simulink library "Blocks"  (R2022b)
settings: Solver=VariableStepAuto  StartTime=0.0  StopTime=10.0  RelTol=1e-3
undefined symbols (not defined in the file): h_send, h_stream_mocap, ID, Payload
libraries: uavmavlinklib x19, dspnetwork x9, hdlsllib x6, $bdroot x6, robotcorelib x2, etargetslib x1, slrealtimeiplib x1
settings Model: Creator=dsor  LastModifiedBy=dsor

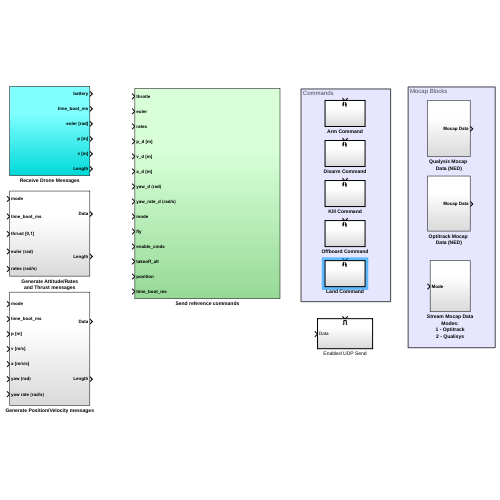
[thumbnail: Simulink's stored preview of the top-level diagram]
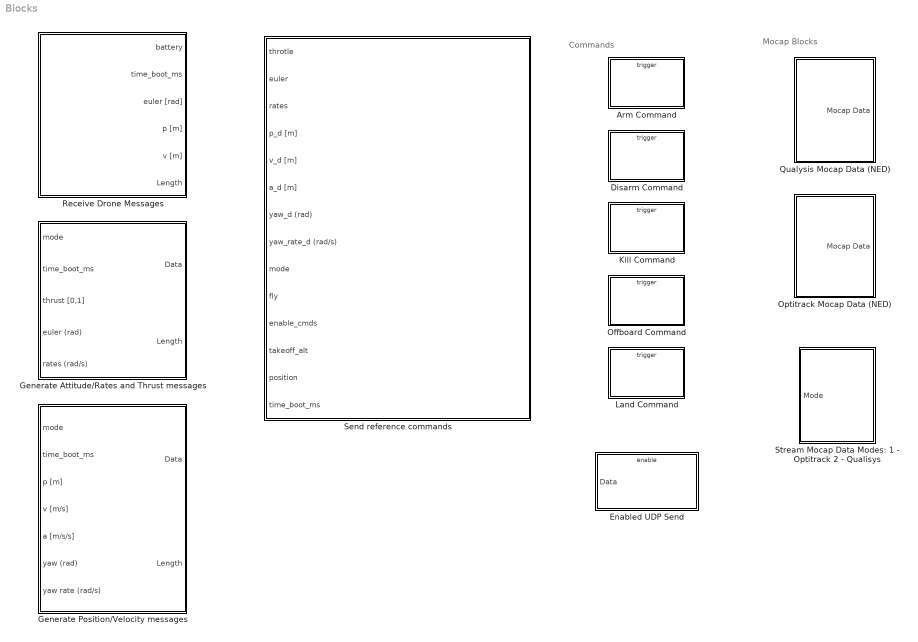
== system Blocks ==
  note: Commands
  note: Mocap Blocks
  Arm Command : Subsystem
  Disarm Command : Subsystem
  Enabled UDP Send : Subsystem
  Generate Attitude/Rates and Thrust messages : Subsystem
  Generate Position/Velocity messages : Subsystem
  Kill Command : Subsystem
  Land Command : Subsystem
  Offboard Command : Subsystem
  Optitrack Mocap Data (NED) : Subsystem
  Qualysis Mocap Data (NED) : Subsystem
  Receive Drone Messages : Subsystem
  Send reference commands : Subsystem
  Stream Mocap Data Modes: 1 - Optitrack 2 - Qualisys : Subsystem

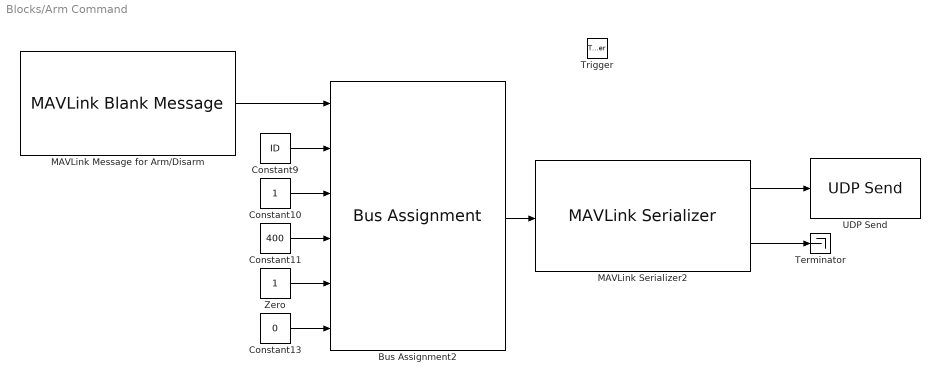
== system Blocks/Arm Command ==
  Trigger : TriggerPort  TriggerType=either  VariantControl=(inherit)  PortDimensions=1
  Bus Assignment2 : BusAssignment  AssignedSignals=Payload.target_system,Payload.target_component,Payload.command,Payload.param1,Payload.param2
  Constant10 : Constant  OutDataTypeStr=uint8
  Constant11 : Constant  Value=400  OutDataTypeStr=uint16
  Constant13 : Constant  Value=0  OutDataTypeStr=single
  Constant9 : Constant  Value=ID  OutDataTypeStr=uint8
  MAVLink Message for Arm/Disarm : uavmavlinklib/MAVLink Blank Message  dialectSource=Select from standard MAVLink dialects  dialect=common.xml  dialectCustom=common.xml  version=2  messageType=COMMAND_LONG  SystemID=255  ComponentID=240  SampleTime=-1
  MAVLink Serializer2 : uavmavlinklib/MAVLink Serializer  dialectSource=Select from standard MAVLink dialects  dialect=common.xml  dialectCustom=common.xml  version=2  messageType=COMMAND_LONG
  Terminator : Terminator
  UDP Send : dspnetwork/UDP Send  remoteURL=Remote_IP  remotePort=Remote_Port  localURL='0.0.0.0'  localPortSource=Specify via dialog  localPort=Local_Port  sendBufferSize=8192  sampletime=-1  blockPlatform=HOST  separateLengthPort=0
      settings: LibrarySourceBlock=embeddedtargetslib/Host Communication/UDP Send
  Zero : Constant  OutDataTypeStr=single
  wires:
  Zero/1 -> Bus Assignment2/5
  MAVLink Serializer2/1 -> UDP Send/1
  MAVLink Message for Arm/Disarm/1 -> Bus Assignment2/1
  Constant9/1 -> Bus Assignment2/2
  Constant13/1 -> Bus Assignment2/6
  Bus Assignment2/1 -> MAVLink Serializer2/1
  Constant10/1 -> Bus Assignment2/3
  Constant11/1 -> Bus Assignment2/4
  MAVLink Serializer2/2 -> Terminator/1

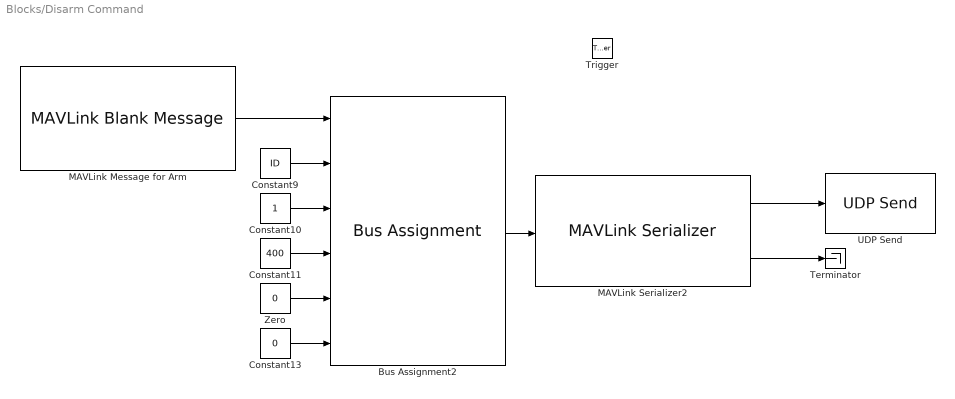
== system Blocks/Disarm Command ==
  Trigger : TriggerPort  TriggerType=either  VariantControl=(inherit)  PortDimensions=1
  Bus Assignment2 : BusAssignment  AssignedSignals=Payload.target_system,Payload.target_component,Payload.command,Payload.param1,Payload.param2
  Constant10 : Constant  OutDataTypeStr=uint8
  Constant11 : Constant  Value=400  OutDataTypeStr=uint16
  Constant13 : Constant  Value=0  OutDataTypeStr=single
  Constant9 : Constant  Value=ID  OutDataTypeStr=uint8
  MAVLink Message for Arm : uavmavlinklib/MAVLink Blank Message  dialectSource=Select from standard MAVLink dialects  dialect=common.xml  dialectCustom=common.xml  version=2  messageType=COMMAND_LONG  SystemID=255  ComponentID=240  SampleTime=-1
  MAVLink Serializer2 : uavmavlinklib/MAVLink Serializer  dialectSource=Select from standard MAVLink dialects  dialect=common.xml  dialectCustom=common.xml  version=2  messageType=COMMAND_LONG
  Terminator : Terminator
  UDP Send : dspnetwork/UDP Send  remoteURL=Remote_IP  remotePort=Remote_Port  localURL='0.0.0.0'  localPortSource=Specify via dialog  localPort=Local_Port  sendBufferSize=8192  sampletime=-1  blockPlatform=HOST  separateLengthPort=0
      settings: LibrarySourceBlock=embeddedtargetslib/Host Communication/UDP Send
  Zero : Constant  Value=0  OutDataTypeStr=single
  wires:
  Zero/1 -> Bus Assignment2/5
  MAVLink Message for Arm/1 -> Bus Assignment2/1
  Constant9/1 -> Bus Assignment2/2
  Constant13/1 -> Bus Assignment2/6
  Bus Assignment2/1 -> MAVLink Serializer2/1
  Constant10/1 -> Bus Assignment2/3
  Constant11/1 -> Bus Assignment2/4
  MAVLink Serializer2/1 -> UDP Send/1
  MAVLink Serializer2/2 -> Terminator/1

== system Blocks/Enabled UDP Send ==
  Data : Inport
  Enable : EnablePort
  UDP Send : dspnetwork/UDP Send  remoteURL=Remote_IP  remotePort=Remote_Port  localURL='0.0.0.0'  localPortSource=Specify via dialog  localPort=Local_Port  sendBufferSize=8192  sampletime=-1  blockPlatform=HOST  separateLengthPort=0
      settings: LibrarySourceBlock=embeddedtargetslib/Host Communication/UDP Send
  wires:
  Data/1 -> UDP Send/1

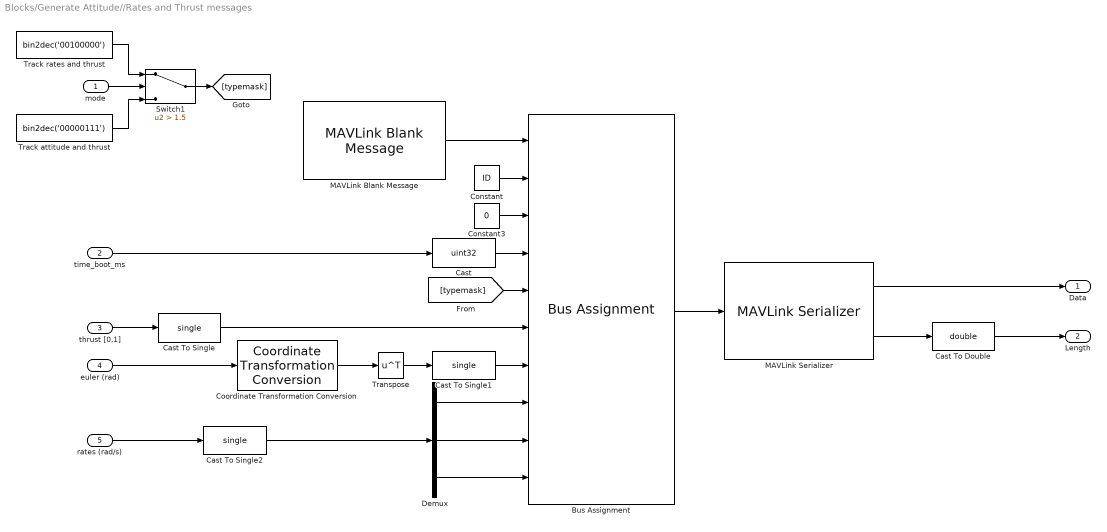
== system Blocks/Generate Attitude//Rates and Thrust messages ==
  mode : Inport  SampleTime=h_send
  time_boot_ms : Inport  Port=2  SampleTime=h_send
  thrust [0,1] : Inport  Port=3  SampleTime=h_send
  euler (rad) : Inport  Port=4  SampleTime=h_send
  rates (rad/s) : Inport  Port=5  SampleTime=h_send
  Bus Assignment : BusAssignment  AssignedSignals=Payload.target_system,Payload.target_component,Payload.time_boot_ms,Payload.type_mask,Payload.thrust,Payload.q,Payload.body_roll_rate,Payload.body_pitch_rate,Payload.body_yaw_rate
  Cast : DataTypeConversion  OutDataTypeStr=uint32  SaturateOnIntegerOverflow=off  RndMeth=Floor
  Cast To Double : DataTypeConversion  OutDataTypeStr=double  SaturateOnIntegerOverflow=off  RndMeth=Floor
  Cast To Single : DataTypeConversion  OutDataTypeStr=single  SaturateOnIntegerOverflow=off  RndMeth=Floor
  Cast To Single1 : DataTypeConversion  OutDataTypeStr=single  SaturateOnIntegerOverflow=off  RndMeth=Floor
  Cast To Single2 : DataTypeConversion  OutDataTypeStr=single  SaturateOnIntegerOverflow=off  RndMeth=Floor
  Constant : Constant  Value=ID  OutDataTypeStr=uint8  SampleTime=h_send
  Constant3 : Constant  Value=0  OutDataTypeStr=uint8  SampleTime=h_send
  Coordinate Transformation Conversion : robotcorelib/Coordinate Transformation Conversion  InputRepresentation=Euler Angles  InputEulerSequence=ZYX  ShowTrVecInputPort=on  OutputRepresentation=Quaternion  OutputEulerSequence=ZYX  ShowTrVecOutputPort=on  SimulateUsing=Interpreted execution
  Demux : Demux  Outputs=3
  MAVLink Blank Message : uavmavlinklib/MAVLink Blank Message  dialectSource=Select from standard MAVLink dialects  dialect=common.xml  dialectCustom=common.xml  version=2  messageType=SET_ATTITUDE_TARGET  SystemID=255  ComponentID=240  SampleTime=h_send
  MAVLink Serializer : uavmavlinklib/MAVLink Serializer  dialectSource=Select from standard MAVLink dialects  dialect=common.xml  dialectCustom=common.xml  version=2  messageType=SET_ATTITUDE_TARGET
  Switch1 : Switch  Criteria=u2 > Threshold  Threshold=1.5  SaturateOnIntegerOverflow=off  InputSameDT=off
  Track attitude and thrust : Constant  Value=bin2dec('00000111')  OutDataTypeStr=uint8  SampleTime=h_send
  Track rates and thrust : Constant  Value=bin2dec('00100000')  OutDataTypeStr=uint8  SampleTime=h_send
  Transpose : Math  Operator=transpose
  Data : Outport  SampleTime=h_send
  Length : Outport  Port=2  SampleTime=h_send
  wires:
  time_boot_ms/1 -> Cast/1
  MAVLink Serializer/2 -> Cast To Double/1
  Cast/1 -> Bus Assignment/4
  Cast To Single1/1 -> Bus Assignment/7
  thrust [0,1]/1 -> Cast To Single/1
  [typemask] -> Bus Assignment/5
  Transpose/1 -> Cast To Single1/1
  Constant3/1 -> Bus Assignment/3
  Constant/1 -> Bus Assignment/2
  MAVLink Blank Message/1 -> Bus Assignment/1
  Cast To Single/1 -> Bus Assignment/6
  Bus Assignment/1 -> MAVLink Serializer/1
  Coordinate Transformation Conversion/1 -> Transpose/1
  euler (rad)/1 -> Coordinate Transformation Conversion/1
  rates (rad/s)/1 -> Cast To Single2/1
  Demux/1 -> Bus Assignment/8
  Demux/2 -> Bus Assignment/9
  Demux/3 -> Bus Assignment/10
  mode/1 -> Switch1/2
  Track rates and thrust/1 -> Switch1/1
  Track attitude and thrust/1 -> Switch1/3
  Switch1/1 -> [typemask]
  Cast To Single2/1 -> Demux/1
  MAVLink Serializer/1 -> Data/1
  Cast To Double/1 -> Length/1

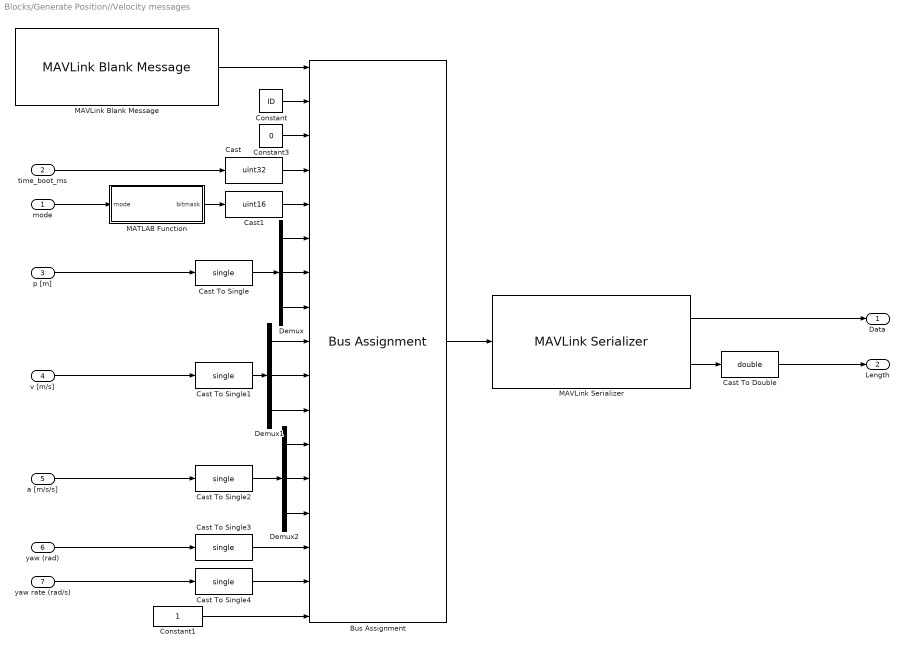
== system Blocks/Generate Position//Velocity messages ==
  mode : Inport  SampleTime=h_send
  time_boot_ms : Inport  Port=2  SampleTime=h_send
  p [m] : Inport  Port=3  SampleTime=h_send
  v [m/s] : Inport  Port=4  SampleTime=h_send
  a [m/s/s] : Inport  Port=5  SampleTime=h_send
  yaw (rad) : Inport  Port=6  SampleTime=h_send
  yaw rate (rad/s) : Inport  Port=7  SampleTime=h_send
  Bus Assignment : BusAssignment  AssignedSignals=Payload.target_system,Payload.target_component,Payload.time_boot_ms,Payload.type_mask,Payload.x,Payload.y,Payload.z,Payload.vx,Payload.vy,Payload.vz,Payload.afx,Payload.afy,Payload.afz,Payload.yaw,Payload.yaw_rate,Payload.coordinate_frame
  Cast : DataTypeConversion  OutDataTypeStr=uint32  SaturateOnIntegerOverflow=off  RndMeth=Floor
  Cast To Double : DataTypeConversion  OutDataTypeStr=double  SaturateOnIntegerOverflow=off  RndMeth=Floor
  Cast To Single{,1..4} (5 alike) : DataTypeConversion  OutDataTypeStr=single  SaturateOnIntegerOverflow=off  RndMeth=Floor
  Cast1 : DataTypeConversion  OutDataTypeStr=uint16  SaturateOnIntegerOverflow=off  RndMeth=Floor
  Constant : Constant  Value=ID  OutDataTypeStr=uint8  SampleTime=h_send
  Constant1 : Constant  OutDataTypeStr=uint8  SampleTime=h_send
  Constant3 : Constant  Value=0  OutDataTypeStr=uint8  SampleTime=h_send
  Demux : Demux  Outputs=3
  Demux1 : Demux  Outputs=3
  Demux2 : Demux  Outputs=3
  MATLAB Function : MATLAB Function  TreatAsAtomicUnit=on
  MAVLink Blank Message : uavmavlinklib/MAVLink Blank Message  dialectSource=Select from standard MAVLink dialects  dialect=common.xml  dialectCustom=common.xml  version=2  messageType=SET_POSITION_TARGET_LOCAL_NED  SystemID=255  ComponentID=240  SampleTime=h_send
  MAVLink Serializer : uavmavlinklib/MAVLink Serializer  dialectSource=Select from standard MAVLink dialects  dialect=common.xml  dialectCustom=common.xml  version=2  messageType=SET_POSITION_TARGET_LOCAL_NED
  Data : Outport  SampleTime=h_send
  Length : Outport  Port=2  SampleTime=h_send
  wires:
  Cast To Single4/1 -> Bus Assignment/16
  Cast1/1 -> Bus Assignment/5
  mode/1 -> MATLAB Function/1(mode)
  yaw rate (rad/s)/1 -> Cast To Single4/1
  Cast To Single3/1 -> Bus Assignment/15
  Cast To Single2/1 -> Demux2/1
  Cast To Single1/1 -> Demux1/1
  Cast To Single/1 -> Demux/1
  Constant1/1 -> Bus Assignment/17
  yaw (rad)/1 -> Cast To Single3/1
  Demux2/1 -> Bus Assignment/12
  Demux2/2 -> Bus Assignment/13
  Demux2/3 -> Bus Assignment/14
  a [m/s/s]/1 -> Cast To Single2/1
  v [m/s]/1 -> Cast To Single1/1
  Demux1/3 -> Bus Assignment/11
  Demux1/2 -> Bus Assignment/10
  Demux1/1 -> Bus Assignment/9
  p [m]/1 -> Cast To Single/1
  Demux/1 -> Bus Assignment/6
  Demux/2 -> Bus Assignment/7
  Demux/3 -> Bus Assignment/8
  Bus Assignment/1 -> MAVLink Serializer/1
  MAVLink Blank Message/1 -> Bus Assignment/1
  Constant/1 -> Bus Assignment/2
  Constant3/1 -> Bus Assignment/3
  MATLAB Function/1(bitmask) -> Cast1/1
  Cast/1 -> Bus Assignment/4
  MAVLink Serializer/2 -> Cast To Double/1
  time_boot_ms/1 -> Cast/1
  MAVLink Serializer/1 -> Data/1
  Cast To Double/1 -> Length/1

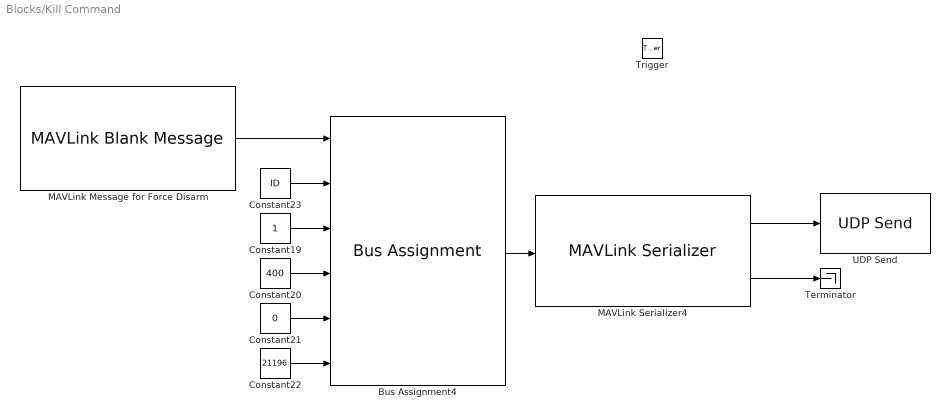
== system Blocks/Kill Command ==
  Trigger : TriggerPort  TriggerType=either  VariantControl=(inherit)  PortDimensions=1
  Bus Assignment4 : BusAssignment  AssignedSignals=Payload.target_system,Payload.target_component,Payload.command,Payload.param1,Payload.param2
  Constant19 : Constant  OutDataTypeStr=uint8
  Constant20 : Constant  Value=400  OutDataTypeStr=uint16
  Constant21 : Constant  Value=0  OutDataTypeStr=single
  Constant22 : Constant  Value=21196  OutDataTypeStr=single
  Constant23 : Constant  Value=ID  OutDataTypeStr=uint8
  MAVLink Message for Force Disarm : uavmavlinklib/MAVLink Blank Message  dialectSource=Select from standard MAVLink dialects  dialect=common.xml  dialectCustom=common.xml  version=2  messageType=COMMAND_LONG  SystemID=255  ComponentID=240  SampleTime=-1
  MAVLink Serializer4 : uavmavlinklib/MAVLink Serializer  dialectSource=Select from standard MAVLink dialects  dialect=common.xml  dialectCustom=common.xml  version=2  messageType=COMMAND_LONG
  Terminator : Terminator
  UDP Send : dspnetwork/UDP Send  remoteURL=Remote_IP  remotePort=Remote_Port  localURL='0.0.0.0'  localPortSource=Specify via dialog  localPort=Local_Port  sendBufferSize=8192  sampletime=-1  blockPlatform=HOST  separateLengthPort=0
      settings: LibrarySourceBlock=embeddedtargetslib/Host Communication/UDP Send
  wires:
  Constant20/1 -> Bus Assignment4/4
  Constant22/1 -> Bus Assignment4/6
  Constant21/1 -> Bus Assignment4/5
  MAVLink Message for Force Disarm/1 -> Bus Assignment4/1
  Bus Assignment4/1 -> MAVLink Serializer4/1
  Constant19/1 -> Bus Assignment4/3
  Constant23/1 -> Bus Assignment4/2
  MAVLink Serializer4/1 -> UDP Send/1
  MAVLink Serializer4/2 -> Terminator/1

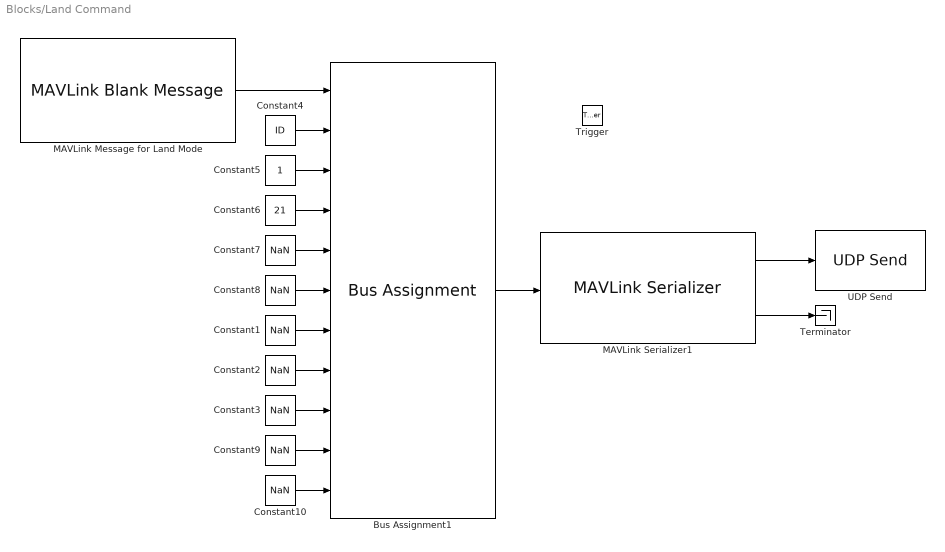
== system Blocks/Land Command ==
  Trigger : TriggerPort  VariantControl=(inherit)  PortDimensions=1
  Bus Assignment1 : BusAssignment  AssignedSignals=Payload.target_system,Payload.target_component,Payload.command,Payload.param1,Payload.param2,Payload.param3,Payload.param4,Payload.param5,Payload.param6,Payload.param7
  Constant{1..3,7..10} (7 alike) : Constant  Value=NaN  OutDataTypeStr=single
  Constant4 : Constant  Value=ID  OutDataTypeStr=uint8
  Constant5 : Constant  OutDataTypeStr=uint8
  Constant6 : Constant  Value=21  OutDataTypeStr=uint16
  MAVLink Message for Land Mode : uavmavlinklib/MAVLink Blank Message  dialectSource=Select from standard MAVLink dialects  dialect=common.xml  dialectCustom=common.xml  version=2  messageType=COMMAND_LONG  SystemID=255  ComponentID=240  SampleTime=-1
  MAVLink Serializer1 : uavmavlinklib/MAVLink Serializer  dialectSource=Select from standard MAVLink dialects  dialect=common.xml  dialectCustom=common.xml  version=2  messageType=COMMAND_LONG
  Terminator : Terminator
  UDP Send : dspnetwork/UDP Send  remoteURL=Remote_IP  remotePort=Remote_Port  localURL='0.0.0.0'  localPortSource=Specify via dialog  localPort=Local_Port  sendBufferSize=8192  sampletime=-1  blockPlatform=HOST  separateLengthPort=0
      settings: LibrarySourceBlock=embeddedtargetslib/Host Communication/UDP Send
  wires:
  Constant4/1 -> Bus Assignment1/2
  Constant8/1 -> Bus Assignment1/6
  Constant6/1 -> Bus Assignment1/4
  Constant5/1 -> Bus Assignment1/3
  MAVLink Message for Land Mode/1 -> Bus Assignment1/1
  Bus Assignment1/1 -> MAVLink Serializer1/1
  Constant7/1 -> Bus Assignment1/5
  Constant10/1 -> Bus Assignment1/11
  Constant9/1 -> Bus Assignment1/10
  Constant3/1 -> Bus Assignment1/9
  Constant2/1 -> Bus Assignment1/8
  Constant1/1 -> Bus Assignment1/7
  MAVLink Serializer1/1 -> UDP Send/1
  MAVLink Serializer1/2 -> Terminator/1

== system Blocks/Offboard Command ==
  Trigger : TriggerPort  TriggerType=either  VariantControl=(inherit)  PortDimensions=1
  Bus Assignment1 : BusAssignment  AssignedSignals=Payload.target_system,Payload.target_component,Payload.command,Payload.param1,Payload.param2
  Constant4 : Constant  Value=ID  OutDataTypeStr=uint8
  Constant5 : Constant  OutDataTypeStr=uint8
  Constant6 : Constant  Value=176  OutDataTypeStr=uint16
  Constant7 : Constant  OutDataTypeStr=single
  Constant8 : Constant  Value=6  OutDataTypeStr=single
  MAVLink Message for Offboard Mode : uavmavlinklib/MAVLink Blank Message  dialectSource=Select from standard MAVLink dialects  dialect=common.xml  dialectCustom=common.xml  version=2  messageType=COMMAND_LONG  SystemID=255  ComponentID=240  SampleTime=-1
  MAVLink Serializer1 : uavmavlinklib/MAVLink Serializer  dialectSource=Select from standard MAVLink dialects  dialect=common.xml  dialectCustom=common.xml  version=2  messageType=COMMAND_LONG
  Terminator : Terminator
  UDP Send : dspnetwork/UDP Send  remoteURL=Remote_IP  remotePort=Remote_Port  localURL='0.0.0.0'  localPortSource=Specify via dialog  localPort=Local_Port  sendBufferSize=8192  sampletime=-1  blockPlatform=HOST  separateLengthPort=0
      settings: LibrarySourceBlock=embeddedtargetslib/Host Communication/UDP Send
  wires:
  Constant7/1 -> Bus Assignment1/5
  Bus Assignment1/1 -> MAVLink Serializer1/1
  MAVLink Message for Offboard Mode/1 -> Bus Assignment1/1
  Constant5/1 -> Bus Assignment1/3
  Constant6/1 -> Bus Assignment1/4
  Constant8/1 -> Bus Assignment1/6
  Constant4/1 -> Bus Assignment1/2
  MAVLink Serializer1/1 -> UDP Send/1
  MAVLink Serializer1/2 -> Terminator/1

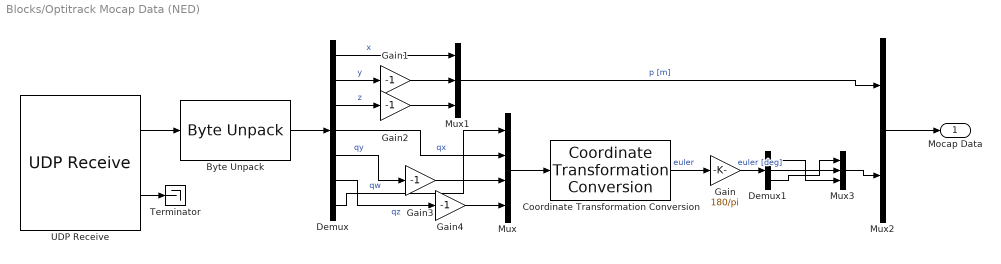
== system Blocks/Optitrack Mocap Data (NED) ==
  Byte Unpack : etargetslib/Byte Unpack  dimensions={[7]}  datatypes={'double'}  byteAlign=4
  Coordinate Transformation Conversion : robotcorelib/Coordinate Transformation Conversion  InputRepresentation=Quaternion  InputEulerSequence=ZYX  ShowTrVecInputPort=on  OutputRepresentation=Euler Angles  OutputEulerSequence=ZYX  ShowTrVecOutputPort=on  SimulateUsing=Interpreted execution
  Demux : Demux  Outputs=7
  Demux1 : Demux  Outputs=3
  Gain : Gain  Gain=180/pi
  Gain{1..4} (4 alike) : Gain  Gain=-1
  Mux : Mux
  Mux1 : Mux  Inputs=3
  Mux2 : Mux  Inputs=2
  Mux3 : Mux  Inputs=3
  Terminator : Terminator
  UDP Receive : dspnetwork/UDP Receive  localURL='0.0.0.0'  localPort=5000  remoteURL='0.0.0.0'  remotePort=-1  recvBufferSize=56  dims=56  signalDatatype=uint8  isComplex=off  isVarSize=off  showBlockingTime=on  blockingTime=0  sampletime=h_optitrack  blockPlatform=HOST
  Mocap Data : Outport
  wires:
  Mux3/1 -> Mux2/2
  Demux1/2 -> Mux3/2
  Demux1/1 -> Mux3/3
  Demux1/3 -> Mux3/1
  Gain/1 -> Demux1/1  "euler [deg]"
  Gain4/1 -> Mux/4
  Gain3/1 -> Mux/3
  Gain2/1 -> Mux1/3
  Gain1/1 -> Mux1/2
  UDP Receive/1 -> Byte Unpack/1
  Demux/3 -> Gain2/1  "z"
  Byte Unpack/1 -> Demux/1
  Demux/1 -> Mux1/1  "x"
  Demux/2 -> Gain1/1  "y"
  UDP Receive/2 -> Terminator/1
  Mux/1 -> Coordinate Transformation Conversion/1
  Mux1/1 -> Mux2/1  "p [m]"
  Mux2/1 -> Mocap Data/1
  Coordinate Transformation Conversion/1 -> Gain/1  "euler"
  Demux/7 -> Mux/1  "qw"
  Demux/4 -> Mux/2  "qx"
  Demux/5 -> Gain3/1  "qy"
  Demux/6 -> Gain4/1  "qz"

== system Blocks/Qualysis Mocap Data (NED) ==
  Constant1 : Constant
  Gain{6..7,9..10} (4 alike) : Gain  Gain=-1
  Mux : Mux  Inputs=6
  Subsystem : Subsystem
  Terminator : Terminator
  UDP Receive1 : dspnetwork/UDP Receive  localURL='0.0.0.0'  localPort=9089  remoteURL='0.0.0.0'  remotePort=-1  recvBufferSize=64  dims=255  signalDatatype=uint8  isComplex=off  isVarSize=off  showBlockingTime=on  blockingTime=0  sampletime=h_qualisys  blockPlatform=HOST
      settings: LibrarySourceBlock=embeddedtargetslib/Host Communication/UDP Receive
  Mocap Data : Outport
  wires:
  Gain6/1 -> Mux/5
  UDP Receive1/2 -> Terminator/1
  Constant1/1 -> Subsystem/2(Object number)
  Subsystem/3(z [m]) -> Gain10/1
  Subsystem/2(y [m]) -> Gain9/1
  UDP Receive1/1 -> Subsystem/1(Data)
  Subsystem/5(pitch [deg]) -> Gain6/1
  Subsystem/6(yaw [deg]) -> Gain7/1
  Gain7/1 -> Mux/6
  Gain10/1 -> Mux/3
  Gain9/1 -> Mux/2
  Subsystem/1(x [m]) -> Mux/1
  Subsystem/4(roll [deg]) -> Mux/4
  Mux/1 -> Mocap Data/1

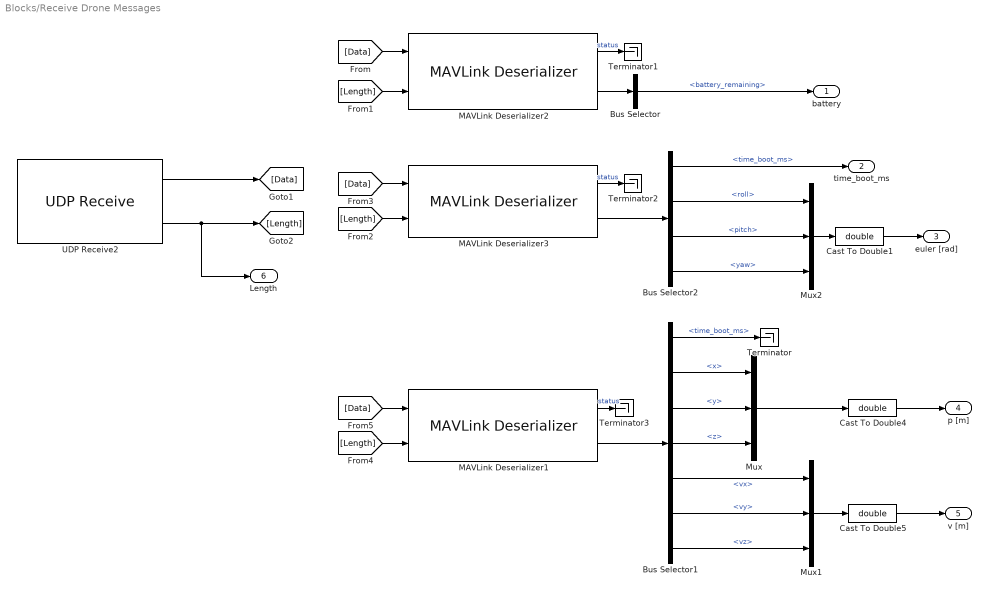
== system Blocks/Receive Drone Messages ==
  Bus Selector : BusSelector  OutputSignals=Payload.battery_remaining
  Bus Selector1 : BusSelector  OutputSignals=Payload.time_boot_ms,Payload.x,Payload.y,Payload.z,Payload.vx,Payload.vy,Payload.vz
  Bus Selector2 : BusSelector  OutputSignals=Payload.time_boot_ms,Payload.roll,Payload.pitch,Payload.yaw
  Cast To Double1 : DataTypeConversion  OutDataTypeStr=double  SaturateOnIntegerOverflow=off  RndMeth=Floor
  Cast To Double4 : DataTypeConversion  OutDataTypeStr=double  SaturateOnIntegerOverflow=off  RndMeth=Floor
  Cast To Double5 : DataTypeConversion  OutDataTypeStr=double  SaturateOnIntegerOverflow=off  RndMeth=Floor
  MAVLink Deserializer1 : uavmavlinklib/MAVLink Deserializer  dialectSource=Select from standard MAVLink dialects  dialect=common.xml  dialectCustom=common.xml  version=2  messageType=LOCAL_POSITION_NED  inputDataLength=on  SystemIDFilter=off  systemID=1  ComponentIDFilter=off  componentID=1  queueMsg=off  queueMsgSize=50  dropNum=off
  MAVLink Deserializer2 : uavmavlinklib/MAVLink Deserializer  dialectSource=Select from standard MAVLink dialects  dialect=common.xml  dialectCustom=common.xml  version=2  messageType=SYS_STATUS  inputDataLength=on  SystemIDFilter=off  systemID=1  ComponentIDFilter=off  componentID=1  queueMsg=off  queueMsgSize=50  dropNum=off
  MAVLink Deserializer3 : uavmavlinklib/MAVLink Deserializer  dialectSource=Select from standard MAVLink dialects  dialect=common.xml  dialectCustom=common.xml  version=2  messageType=ATTITUDE  inputDataLength=on  SystemIDFilter=off  systemID=1  ComponentIDFilter=off  componentID=1  queueMsg=off  queueMsgSize=50  dropNum=off
  Mux : Mux  Inputs=3
  Mux1 : Mux  Inputs=3
  Mux2 : Mux  Inputs=3
  Terminator{,1..3} (4 alike) : Terminator
  UDP Receive2 : dspnetwork/UDP Receive  localURL='0.0.0.0'  localPort=Local_Port  remoteURL='0.0.0.0'  remotePort=-1  recvBufferSize=8192  dims=255  signalDatatype=uint8  isComplex=off  isVarSize=off  showBlockingTime=on  blockingTime=0  sampletime=h_receive  blockPlatform=HOST
      settings: LibrarySourceBlock=embeddedtargetslib/Host Communication/UDP Receive
  battery : Outport
  time_boot_ms : Outport  Port=2
  euler [rad] : Outport  Port=3
  p [m] : Outport  Port=4
  v [m] : Outport  Port=5
  Length : Outport  Port=6
  wires:
  Mux1/1 -> Cast To Double5/1
  Cast To Double4/1 -> p [m]/1
  [Length] -> MAVLink Deserializer1/2
  Cast To Double5/1 -> v [m]/1
  Bus Selector1/6 -> Mux1/2  "<vy>"
  Bus Selector1/3 -> Mux/2  "<y>"
  Bus Selector1/1 -> Terminator/1  "<time_boot_ms>"
  Mux/1 -> Cast To Double4/1
  [Length] -> MAVLink Deserializer3/2
  Bus Selector1/2 -> Mux/1  "<x>"
  Bus Selector2/1 -> time_boot_ms/1  "<time_boot_ms>"
  [Data] -> MAVLink Deserializer3/1
  MAVLink Deserializer1/2 -> Bus Selector1/1
  Bus Selector1/7 -> Mux1/3  "<vz>"
  Bus Selector/1 -> battery/1  "<battery_remaining>"
  [Data] -> MAVLink Deserializer1/1
  [Data] -> MAVLink Deserializer2/1
  Bus Selector2/2 -> Mux2/1  "<roll>"
  Mux2/1 -> Cast To Double1/1
  MAVLink Deserializer1/1 -> Terminator3/1  "status"
  Bus Selector2/4 -> Mux2/3  "<yaw>"
  Bus Selector1/5 -> Mux1/1  "<vx>"
  Bus Selector2/3 -> Mux2/2  "<pitch>"
  MAVLink Deserializer2/1 -> Terminator1/1  "status"
  [Length] -> MAVLink Deserializer2/2
  MAVLink Deserializer3/2 -> Bus Selector2/1
  Bus Selector1/4 -> Mux/3  "<z>"
  MAVLink Deserializer2/2 -> Bus Selector/1
  Cast To Double1/1 -> euler [rad]/1
  MAVLink Deserializer3/1 -> Terminator2/1  "status"
  UDP Receive2/2 -> Length/1, [Length]
  UDP Receive2/1 -> [Data]

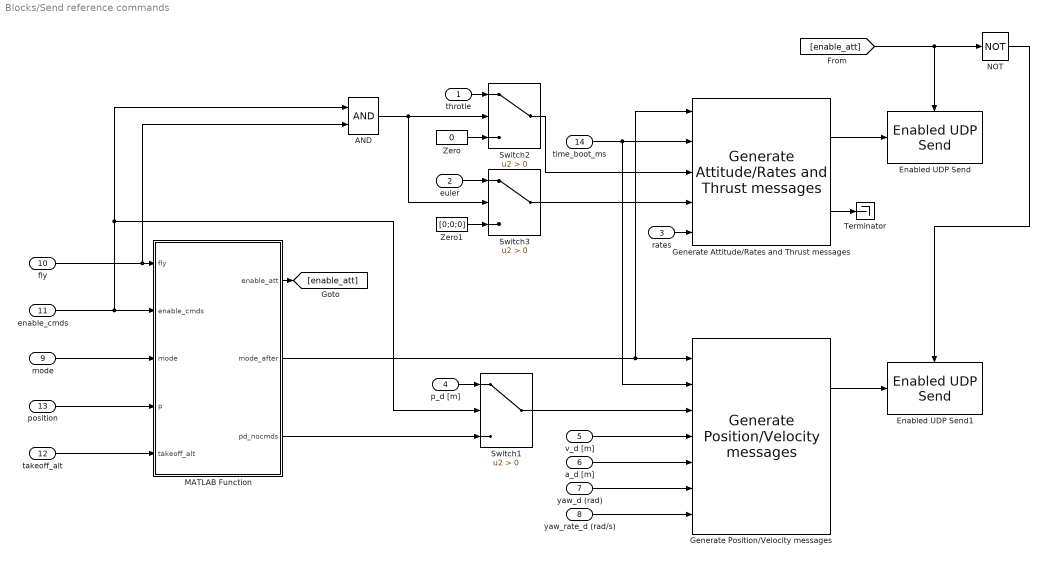
== system Blocks/Send reference commands ==
  throtle : Inport  SampleTime=h_send
  euler : Inport  Port=2  SampleTime=h_send
  rates : Inport  Port=3  SampleTime=h_send
  p_d [m] : Inport  Port=4  SampleTime=h_send
  v_d [m] : Inport  Port=5  SampleTime=h_send
  a_d [m] : Inport  Port=6  SampleTime=h_send
  yaw_d (rad) : Inport  Port=7  SampleTime=h_send
  yaw_rate_d (rad/s) : Inport  Port=8  SampleTime=h_send
  mode : Inport  Port=9  SampleTime=h_send
  fly : Inport  Port=10  SampleTime=h_send
  enable_cmds : Inport  Port=11  SampleTime=h_send
  takeoff_alt : Inport  Port=12  SampleTime=h_send
  position : Inport  Port=13  SampleTime=h_send
  time_boot_ms : Inport  Port=14  SampleTime=h_send
  AND : Logic  IconShape=distinctive  AllPortsSameDT=off  OutDataTypeStr=boolean
  Enabled UDP Send : $bdroot/Enabled UDP Send  SystemSampleTime=-1  VariantActivationTime=update diagram  Latency=0  AutoFrameSizeCalculation=off
  Enabled UDP Send1 : $bdroot/Enabled UDP Send  SystemSampleTime=-1  VariantActivationTime=update diagram  Latency=0  AutoFrameSizeCalculation=off
  Generate Attitude/Rates and Thrust messages : $bdroot/Generate Attitude//Rates and Thrust messages  SystemSampleTime=-1  VariantActivationTime=update diagram  Latency=0  AutoFrameSizeCalculation=off
  Generate Position/Velocity messages : $bdroot/Generate Position//Velocity messages  SystemSampleTime=-1  VariantActivationTime=update diagram  Latency=0  AutoFrameSizeCalculation=off
  MATLAB Function : MATLAB Function  TreatAsAtomicUnit=on
  NOT : Logic  Operator=NOT  IconShape=distinctive  AllPortsSameDT=off  OutDataTypeStr=boolean
  Switch1 : Switch  Criteria=u2 > Threshold  SaturateOnIntegerOverflow=off  InputSameDT=off
  Switch2 : Switch  Criteria=u2 > Threshold  SaturateOnIntegerOverflow=off  InputSameDT=off
  Switch3 : Switch  Criteria=u2 > Threshold  SaturateOnIntegerOverflow=off  InputSameDT=off
  Terminator : Terminator
  Zero : Constant  Value=0  OutDataTypeStr=Inherit: Inherit via back propagation
  Zero1 : Constant  Value=[0;0;0]  OutDataTypeStr=Inherit: Inherit via back propagation
  wires:
  v_d [m]/1 -> Generate Position/Velocity messages/4
  throtle/1 -> Switch2/1
  position/1 -> MATLAB Function/4(p)
  p_d [m]/1 -> Switch1/1
  Switch1/1 -> Generate Position/Velocity messages/3
  yaw_d (rad)/1 -> Generate Position/Velocity messages/6
  a_d [m]/1 -> Generate Position/Velocity messages/5
  Zero1/1 -> Switch3/3
  Switch3/1 -> Generate Attitude/Rates and Thrust messages/4
  enable_cmds/1 -> Switch1/2, AND/1, MATLAB Function/2(enable_cmds)
  MATLAB Function/2(mode_after) -> Generate Attitude/Rates and Thrust messages/1, Generate Position/Velocity messages/1
  Switch2/1 -> Generate Attitude/Rates and Thrust messages/3
  AND/1 -> Switch3/2, Switch2/2
  MATLAB Function/3(pd_nocmds) -> Switch1/3
  rates/1 -> Generate Attitude/Rates and Thrust messages/5
  yaw_rate_d (rad/s)/1 -> Generate Position/Velocity messages/7
  time_boot_ms/1 -> Generate Attitude/Rates and Thrust messages/2, Generate Position/Velocity messages/2
  fly/1 -> AND/2, MATLAB Function/1(fly)
  mode/1 -> MATLAB Function/3(mode)
  euler/1 -> Switch3/1
  Zero/1 -> Switch2/3
  takeoff_alt/1 -> MATLAB Function/5(takeoff_alt)
  Generate Attitude/Rates and Thrust messages/1 -> Enabled UDP Send/1
  Generate Attitude/Rates and Thrust messages/2 -> Terminator/1
  Generate Position/Velocity messages/1 -> Enabled UDP Send1/1
  MATLAB Function/1(enable_att) -> [enable_att]
  [enable_att] -> NOT/1, Enabled UDP Send/Enable
  NOT/1 -> Enabled UDP Send1/Enable

== system Blocks/Stream Mocap Data Modes: 1 - Optitrack 2 - Qualisys ==
  note: Modes
      | 0 - Disable
      | 1 - Optitrack
      | 2 - Qualisys
  Mode : Inport
  Optitrack Mocap Data (NED) : $bdroot/Optitrack Mocap  Data (NED)  SystemSampleTime=-1  VariantActivationTime=update diagram  Latency=0  AutoFrameSizeCalculation=off
  Qualysis Mocap Data (NED) : $bdroot/Qualysis Mocap  Data (NED)  SystemSampleTime=-1  VariantActivationTime=update diagram  Latency=0  AutoFrameSizeCalculation=off
  Rate Transition : RateTransition  OutPortSampleTime=h_stream_mocap
  Rate Transition1 : RateTransition  OutPortSampleTime=h_stream_mocap
  Stream Mocap Data to the Drone (must be in NED) : Subsystem
  Switch : Switch  Criteria=u2 > Threshold  Threshold=1.5  SaturateOnIntegerOverflow=off  InputSameDT=off
  wires:
  Switch/1 -> Stream Mocap Data to the Drone (must be in NED)/2(Mocap Data)
  Optitrack Mocap Data (NED)/1 -> Rate Transition1/1
  Qualysis Mocap Data (NED)/1 -> Rate Transition/1
  Rate Transition/1 -> Switch/1
  Mode/1 -> Stream Mocap Data to the Drone (must be in NED)/1(enable), Switch/2
  Rate Transition1/1 -> Switch/3

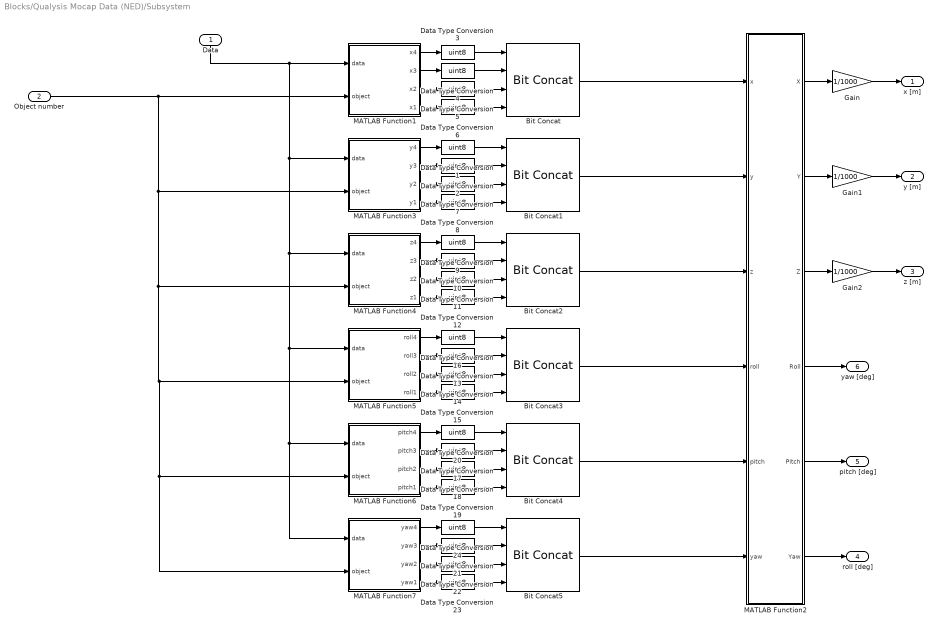
== system Blocks/Qualysis Mocap Data (NED)/Subsystem ==
  Data : Inport
  Object number : Inport  Port=2
  Bit Concat{,1..5} (6 alike) : hdlsllib/Logic and Bit Operations/Bit Concat  numInputs=4
  Data Type Conversion{1..24} (24 alike) : DataTypeConversion  OutDataTypeStr=uint8  SaturateOnIntegerOverflow=off  RndMeth=Floor
  Gain : Gain  Gain=1/1000
  Gain1 : Gain  Gain=1/1000
  Gain2 : Gain  Gain=1/1000
  MATLAB Function1 : MATLAB Function  TreatAsAtomicUnit=on
  MATLAB Function2 : MATLAB Function  TreatAsAtomicUnit=on
  MATLAB Function3 : MATLAB Function  TreatAsAtomicUnit=on
  MATLAB Function4 : MATLAB Function  TreatAsAtomicUnit=on
  MATLAB Function5 : MATLAB Function  TreatAsAtomicUnit=on
  MATLAB Function6 : MATLAB Function  TreatAsAtomicUnit=on
  MATLAB Function7 : MATLAB Function  TreatAsAtomicUnit=on
  x [m] : Outport  VectorParamsAs1DForOutWhenUnconnected=off
  y [m] : Outport  Port=2  VectorParamsAs1DForOutWhenUnconnected=off
  z [m] : Outport  Port=3  VectorParamsAs1DForOutWhenUnconnected=off
  roll [deg] : Outport  Port=4  VectorParamsAs1DForOutWhenUnconnected=off
  pitch [deg] : Outport  Port=5  VectorParamsAs1DForOutWhenUnconnected=off
  yaw [deg] : Outport  Port=6  VectorParamsAs1DForOutWhenUnconnected=off
  wires:
  Data Type Conversion6/1 -> Bit Concat/4
  Data Type Conversion3/1 -> Bit Concat/1
  MATLAB Function1/3(x2) -> Data Type Conversion5/1
  MATLAB Function2/1(X) -> Gain/1
  MATLAB Function4/1(z4) -> Data Type Conversion9/1
  MATLAB Function4/2(z3) -> Data Type Conversion10/1
  Bit Concat2/1 -> MATLAB Function2/3(z)
  Data Type Conversion12/1 -> Bit Concat2/4
  Data Type Conversion11/1 -> Bit Concat2/3
  MATLAB Function4/4(z1) -> Data Type Conversion12/1
  Data Type Conversion10/1 -> Bit Concat2/2
  MATLAB Function4/3(z2) -> Data Type Conversion11/1
  Data Type Conversion9/1 -> Bit Concat2/1
  MATLAB Function2/5(Pitch) -> pitch [deg]/1
  MATLAB Function2/2(Y) -> Gain1/1
  MATLAB Function2/6(Yaw) -> roll [deg]/1
  Data Type Conversion14/1 -> Bit Concat3/3
  MATLAB Function5/3(roll2) -> Data Type Conversion14/1
  Bit Concat3/1 -> MATLAB Function2/4(roll)
  MATLAB Function5/2(roll3) -> Data Type Conversion13/1
  Data Type Conversion13/1 -> Bit Concat3/2
  Data Type Conversion15/1 -> Bit Concat3/4
  Data Type Conversion16/1 -> Bit Concat3/1
  MATLAB Function5/1(roll4) -> Data Type Conversion16/1
  MATLAB Function5/4(roll1) -> Data Type Conversion15/1
  MATLAB Function1/2(x3) -> Data Type Conversion4/1
  MATLAB Function1/4(x1) -> Data Type Conversion6/1
  MATLAB Function1/1(x4) -> Data Type Conversion3/1
  Bit Concat/1 -> MATLAB Function2/1(x)
  MATLAB Function2/3(Z) -> Gain2/1
  MATLAB Function2/4(Roll) -> yaw [deg]/1
  Data Type Conversion5/1 -> Bit Concat/3
  Data/1 -> MATLAB Function1/1(data), MATLAB Function7/1(data), MATLAB Function6/1(data), MATLAB Function5/1(data), MATLAB Function4/1(data), MATLAB Function3/1(data)
  Data Type Conversion4/1 -> Bit Concat/2
  Data Type Conversion20/1 -> Bit Concat4/1
  MATLAB Function6/2(pitch3) -> Data Type Conversion17/1
  MATLAB Function6/3(pitch2) -> Data Type Conversion18/1
  Data Type Conversion17/1 -> Bit Concat4/2
  MATLAB Function6/1(pitch4) -> Data Type Conversion20/1
  Data Type Conversion19/1 -> Bit Concat4/4
  MATLAB Function6/4(pitch1) -> Data Type Conversion19/1
  Bit Concat4/1 -> MATLAB Function2/5(pitch)
  Data Type Conversion18/1 -> Bit Concat4/3
  MATLAB Function7/1(yaw4) -> Data Type Conversion24/1
  Bit Concat5/1 -> MATLAB Function2/6(yaw)
  Data Type Conversion24/1 -> Bit Concat5/1
  Data Type Conversion22/1 -> Bit Concat5/3
  MATLAB Function7/3(yaw2) -> Data Type Conversion22/1
  Data Type Conversion21/1 -> Bit Concat5/2
  Object number/1 -> MATLAB Function1/2(object), MATLAB Function7/2(object), MATLAB Function6/2(object), MATLAB Function5/2(object), MATLAB Function4/2(object), MATLAB Function3/2(object)
  MATLAB Function7/4(yaw1) -> Data Type Conversion23/1
  Data Type Conversion23/1 -> Bit Concat5/4
  MATLAB Function7/2(yaw3) -> Data Type Conversion21/1
  MATLAB Function3/1(y4) -> Data Type Conversion1/1
  MATLAB Function3/3(y2) -> Data Type Conversion7/1
  Data Type Conversion8/1 -> Bit Concat1/4
  Data Type Conversion2/1 -> Bit Concat1/2
  MATLAB Function3/4(y1) -> Data Type Conversion8/1
  MATLAB Function3/2(y3) -> Data Type Conversion2/1
  Data Type Conversion1/1 -> Bit Concat1/1
  Bit Concat1/1 -> MATLAB Function2/2(y)
  Data Type Conversion7/1 -> Bit Concat1/3
  Gain/1 -> x [m]/1
  Gain1/1 -> y [m]/1
  Gain2/1 -> z [m]/1

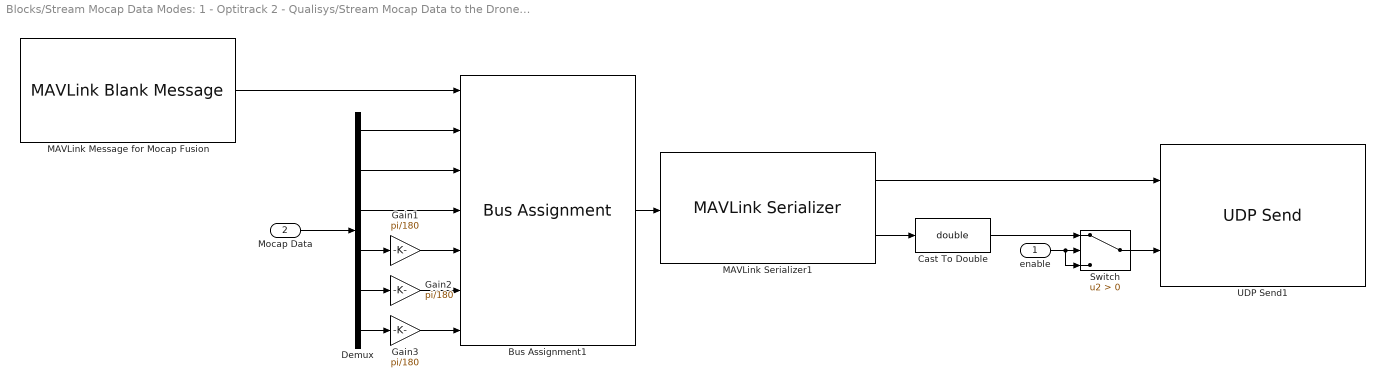
== system Blocks/Stream Mocap Data Modes: 1 - Optitrack 2 - Qualisys/Stream Mocap Data to the Drone (must be in NED) ==
  enable : Inport
  Mocap Data : Inport  Port=2  SampleTime=h_stream_mocap
  Bus Assignment1 : BusAssignment  AssignedSignals=Payload.x,Payload.y,Payload.z,Payload.roll,Payload.pitch,Payload.yaw
  Cast To Double : DataTypeConversion  OutDataTypeStr=double  SaturateOnIntegerOverflow=off  RndMeth=Floor
  Demux : Demux  Outputs=6
  Gain1 : Gain  Gain=pi/180
  Gain2 : Gain  Gain=pi/180
  Gain3 : Gain  Gain=pi/180
  MAVLink Message for Mocap Fusion : uavmavlinklib/MAVLink Blank Message  dialectSource=Select from standard MAVLink dialects  dialect=common.xml  dialectCustom=common.xml  version=2  messageType=VISION_POSITION_ESTIMATE  SystemID=255  ComponentID=240  SampleTime=h_stream_mocap
  MAVLink Serializer1 : uavmavlinklib/MAVLink Serializer  dialectSource=Select from standard MAVLink dialects  dialect=common.xml  dialectCustom=common.xml  version=2  messageType=VISION_POSITION_ESTIMATE
  Switch : Switch  Criteria=u2 > Threshold  SaturateOnIntegerOverflow=off  InputSameDT=off
  UDP Send1 : slrealtimeiplib/UDP Send  useHostTargetConn=off  toAddress=Remote_IP  toPort=Remote_Port  sampleTime=h_stream_mocap  enableMessage=off  ipAddress=Local_IP  localPort=10000
  wires:
  MAVLink Serializer1/1 -> UDP Send1/1
  MAVLink Message for Mocap Fusion/1 -> Bus Assignment1/1
  Bus Assignment1/1 -> MAVLink Serializer1/1
  MAVLink Serializer1/2 -> Cast To Double/1
  Gain3/1 -> Bus Assignment1/7
  Gain2/1 -> Bus Assignment1/6
  Gain1/1 -> Bus Assignment1/5
  Mocap Data/1 -> Demux/1
  Demux/4 -> Gain1/1
  Demux/5 -> Gain2/1
  Demux/6 -> Gain3/1
  Demux/3 -> Bus Assignment1/4
  Demux/2 -> Bus Assignment1/3
  Demux/1 -> Bus Assignment1/2
  Cast To Double/1 -> Switch/1
  Switch/1 -> UDP Send1/2
  enable/1 -> Switch/3, Switch/2

== matlab function Blocks/Qualysis Mocap Data (NED)/Subsystem/MATLAB Function6 ==
  data: pitch4 output uint8; pitch3 output uint8; pitch2 output uint8; data input; pitch1 output uint8; object input
function [pitch4,pitch3,pitch2,pitch1] = fcn(data,object)

slot=(object-1)*8;

pitch1=data(57+slot);
pitch2=data(57+slot+1);
pitch3=data(57+slot+2);
pitch4=data(57+slot+3);

== matlab function Blocks/Qualysis Mocap Data (NED)/Subsystem/MATLAB Function7 ==
  data: yaw4 output uint8; yaw3 output uint8; yaw2 output uint8; data input; yaw1 output uint8; object input
function [yaw4,yaw3,yaw2,yaw1] = fcn(data,object)

slot=(object-1)*8;

yaw1=data(61+slot);
yaw2=data(61+slot+1);
yaw3=data(61+slot+2);
yaw4=data(61+slot+3);

== matlab function Blocks/Send reference commands/MATLAB Function ==
  data: fly input; enable_cmds input; mode input; enable_att output; mode_after output; p input; pd_nocmds output; takeoff_alt input
function [enable_att,mode_after,pd_nocmds] = ModelLogic(fly, enable_cmds, mode, p, takeoff_alt)
    
    %% Persistent variables initialization
    persistent pd
    persistent fly_previous
    persistent enable_cmds_previous
    if isempty(pd)
        pd = [0,0,0];
        fly_previous = 0;
        enable_cmds_previous = 0;
    end


    %% Position is received as a column vector and the function works with line vector.
    p = p';     

    %% Logic to prepare commands to send
    if fly == 1
        if enable_cmds == 0 && enable_cmds_previous == 0        % Hold mode
            enable_att = 0;
            mode_after = 3;
        elseif enable_cmds == 0 && enable_cmds_previous == 1    % Start hold at current position
            enable_att = 0;
            mode_after = 3;
            pd = p;
        else    % enable_cmds == 1 - Send user commands
            mode_after = mode;
            if mode <= 2
                enable_att = 1;
            else
                enable_att = 0;
            end
        end
    else
        enable_att = 1;
        mode_after = 1;
    end

    %% Do special actions when landing or takeoff are triggered.
    if fly_previous == 0 && fly == 1
        enable_att = 0;
        pd = p + [0,0,-takeoff_alt];
        mode_after = 3;
    elseif fly_previous == 1 && fly == 0
        enable_att = 1;
        mode_after = 1;
        pd = p;
    end

    %% Update variables to send
    enable_cmds_previous = enable_cmds;
    pd_nocmds = pd(1:3);
    fly_previous = fly;

end

== matlab function Blocks/Generate Position//Velocity messages/MATLAB Function ==
  data: mode input; bitmask output
function bitmask = fcn(mode)
    bitmask = bin2dec('100111111000');    
    if mode == 3
        bitmask = bin2dec('100111111000');
    else
        bitmask = bin2dec('100111111000');
    end

== matlab function Blocks/Qualysis Mocap Data (NED)/Subsystem/MATLAB Function1 ==
  data: x4 output uint8; x3 output uint8; x2 output uint8; data input; x1 output uint8; object input
function [x4,x3,x2,x1] = fcn(data,object)

slot=(object-1)*8;

x1=data(41+slot);
x2=data(41+slot+1);
x3=data(41+slot+2);
x4=data(41+slot+3);

== matlab function Blocks/Qualysis Mocap Data (NED)/Subsystem/MATLAB Function2 ==
  data: x input uint32 size=1; X output single size=1; y input; Y output; z input; roll input; pitch input; yaw input; Z output; Roll output; Pitch output; Yaw output
function [X,Y,Z,Roll,Pitch,Yaw] = fcn(x,y,z,roll,pitch,yaw)


X = typecast(uint32(x),'single');
Y = typecast(uint32(y),'single');
Z = typecast(uint32(z),'single');
Roll = typecast(uint32(roll),'single');
Pitch = typecast(uint32(pitch),'single');
Yaw = typecast(uint32(yaw),'single');

== matlab function Blocks/Qualysis Mocap Data (NED)/Subsystem/MATLAB Function3 ==
  data: y4 output uint8; y3 output uint8; y2 output uint8; data input; y1 output uint8; object input
function [y4,y3,y2,y1] = fcn(data,object)

slot=(object-1)*8;

y1=data(45+slot);
y2=data(45+slot+1);
y3=data(45+slot+2);
y4=data(45+slot+3);

== matlab function Blocks/Qualysis Mocap Data (NED)/Subsystem/MATLAB Function4 ==
  data: z4 output uint8; z3 output uint8; z2 output uint8; data input; z1 output uint8; object input
function [z4,z3,z2,z1] = fcn(data,object)

slot=(object-1)*8;

z1=data(49+slot);
z2=data(49+slot+1);
z3=data(49+slot+2);
z4=data(49+slot+3);

== matlab function Blocks/Qualysis Mocap Data (NED)/Subsystem/MATLAB Function5 ==
  data: roll4 output uint8; roll3 output uint8; roll2 output uint8; data input; roll1 output uint8; object input
function [roll4,roll3,roll2,roll1] = fcn(data,object)

slot=(object-1)*8;

roll1=data(53+slot);
roll2=data(53+slot+1);
roll3=data(53+slot+2);
roll4=data(53+slot+3);
